simulink model "Controllo_LQ_int"  (R2023b)
settings: Solver=ode45  StartTime=0.0  StopTime=20  MaxStep=0.005  RelTol=1e-3  EnableMultiTasking=on
undefined symbols (not defined in the file): A, B, C, C_add, D, Kint1, Kint2
settings Model: Creator=roberto  LastModifiedBy=roberto_ambrosino
settings SolverCC: AlgebraicLoopSolver=TrustRegion
settings DataIOCC: LimitDataPoints=on  SaveFormat=Array  ReturnWorkspaceOutputs=off
settings OptimizationCC: LifeSpan=inf
settings DebuggingCC: UnconnectedInputMsg=warning  UnconnectedOutputMsg=warning  UnconnectedLineMsg=warning  SFUnexpectedBacktrackingDiag=warning  SFNoUnconditionalDefaultTransitionDiag=warning  SFExecutionAtInitializationDiag=none  ArithmeticOperatorsInVariantConditions=warning
settings HardwareCC: ProdBitPerPointer=32  ProdBitPerSizeT=32  ProdBitPerPtrDiffT=32  ProdLargestAtomicFloat=None  ProdIntDivRoundTo=Undefined  ProdEndianess=Unspecified  ProdWordSize=32  ProdHWDeviceType=32-bit Generic
settings ModelReferenceCC: EnableRefExpFcnMdlSchedulingChecks=on  PropagateSignalLabelsOutOfModel=off
settings SFSimCC: SimUseLocalCustomCode=off  CustomCodeUndefinedFunction=UseInterfaceOnly
settings RTWCC: RTWUseLocalCustomCode=off  DLArmComputeVersion=19.05
settings CodeAppCC: StateflowObjectComments=on
settings GRTTargetCC: TargetLangStandard=C89/C90 (ANSI)
settings ConfigComp: CovMetricSettings=dw  CovSaveCumulativeToWorkspaceVar=on  CovSaveSingleToWorkspaceVar=on  CovExternalEMLEnable=off

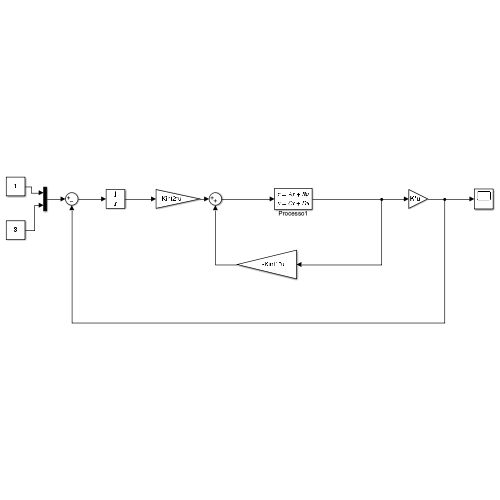
[thumbnail: Simulink's stored preview of the top-level diagram]
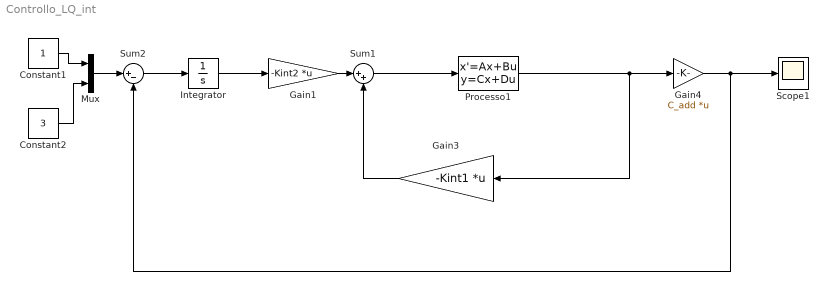
== system Controllo_LQ_int ==
  Constant1 : Constant
  Constant2 : Constant  Value=3
  Gain1 : Gain  Gain=-Kint2  Multiplication=Matrix(K*u)
  Gain3 : Gain  Gain=-Kint1  Multiplication=Matrix(K*u)
  Gain4 : Gain  Gain=C_add  Multiplication=Matrix(K*u)
  Integrator : Integrator
  Mux : Mux  Inputs=2
  Processo1 : StateSpace  A=A  B=B  C=C  D=D  InitialCondition=[0 0 2 0 4 0]
  Scope1 : Scope
  Sum1 : Sum  Inputs=|++
  Sum2 : Sum  Inputs=|+-
  wires:
  Processo1/1 -> Gain3/1, Gain4/1
  Sum1/1 -> Processo1/1
  Gain4/1 -> Sum2/2, Scope1/1
  Gain3/1 -> Sum1/2
  Sum2/1 -> Integrator/1
  Integrator/1 -> Gain1/1
  Gain1/1 -> Sum1/1
  Mux/1 -> Sum2/1
  Constant1/1 -> Mux/1
  Constant2/1 -> Mux/2
